simulink model "xpcserialbinarytest"  (Simulink 7.1)
settings: Solver=FixedStepDiscrete  StartTime=0.0  StopTime=inf  RelTol=1e-3
InitFcn:
  | trun = .1;
values from neighbouring files (symbols this model uses):
  count = count+1    (= 2)    [findVI.m]
undefined symbols (not defined in the file or in its folder): mquafifomask
libraries: xpclib x78, simulink x3
Description:
  | Serial Blocks Loopback Test Using Binary Encoding/Decoding
  | 
  | This model demonstrates the BINARY FIFO read block in a form that can be simulated without using any specific serial hardware.  The input to the FIFO write block is the concatenation of several pieces comprising two separate 'messages'.  The first message is the byte stream: [170, 1, N] and the second is [170 2 44 M] where N is an incrementing number and M is a decrementing number.  The initial '8' in the first constant is the number of elements that follow.  The '5' is an extraneous value that shows how the FIFO binary read will ignore extra information.
  | 
  | To run this test with real serial port hardware, replace the FIFO write block with the send/receive block with FIFO OUT that corresponds to your hardware from the xpclib rs232 section. Then feed the output signal back to the input with a wire to perform a loopback test.
settings Model: Creator=gweast  LastModifiedBy=Administrator  ExtModeArmWhenConnect=off  BufferReuse=off
settings OptimizationCC: BlockReduction=off  OptimizeBlockIOStorage=off  BufferReuse=off  ExpressionFolding=off  FoldNonRolledExpr=off  LocalBlockOutputs=off
settings DebuggingCC: SaveWithParameterizedLinksMsg=none  SignalResolutionControl=TryResolveAllWithWarning  MultiTaskDSMMsg=warning  MultiTaskCondExecSysMsg=none  StrictBusMsg=None
settings HardwareCC: ProdIntDivRoundTo=Zero  ProdEndianess=LittleEndian  ProdHWDeviceType=Generic->32-bit x86 compatible
settings RTWCC: SystemTargetFile=xpctarget.tlc  TemplateMakefile=xpc_default_tmf  Description=xPC Target  ProcessScript=xpctarget_make_rtw_hook  IncludeERTFirstTime=on
settings xpcTargetCC: TargetFcnLib=ansi_tfl_tmw.mat  TargetFunctionLibrary=ANSI_C  CompOptLevelCompliant=off  PortableWordSizes=off  xPCisDownloadable=off

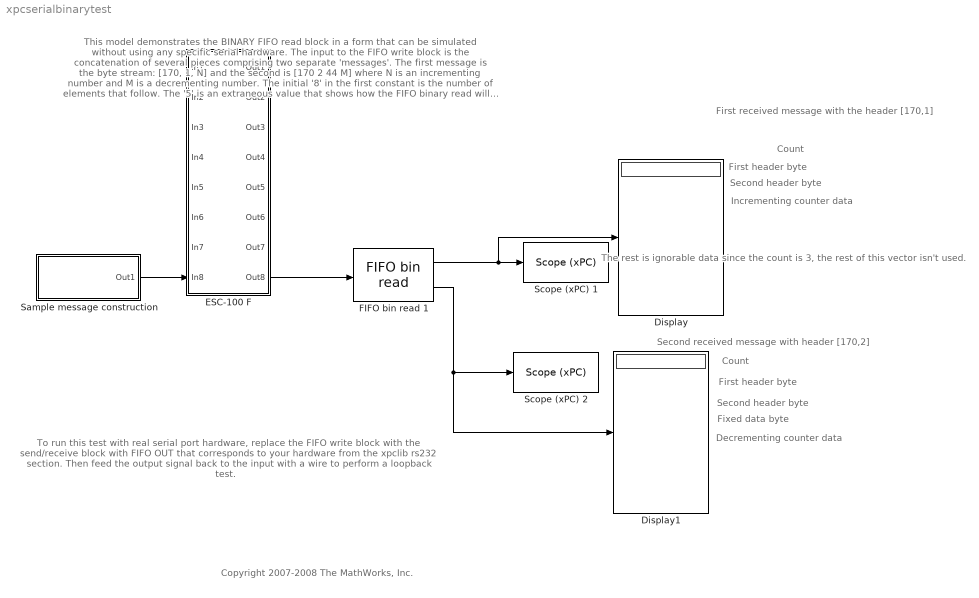
== system xpcserialbinarytest ==
  note: This model demonstrates the BINARY FIFO read block in a form that can
      | be simulated without using any specific serial hardware.  The input to
      | the FIFO write block is the concatenation of several pieces comprising
      | two separate 'messages'.  The first message is the byte stream:
      | [170, 1, N] and the second is [170 2 44 M] where N is an incrementing
      | number and M is a decrementing number.  The initial '8' in the first constant
      | is the number of elements that follow.  The '5' is an extraneous value that
      | shows how the FIFO binary read will ignore extra information.
  note: To run this test with
      | real serial port hardware,
      | replace the FIFO write
      | block with the send/receive
      | block with FIFO OUT that
      | corresponds to your
      | hardware from the xpclib
      | rs232 section. Then feed
      | the output signal back to
      | the input with a wire to
      | perform a loopback test.
  note: First received message
      | with the header [170,1]
  note: Count
  note: First header byte
  note: Second header byte
  note: Incrementing counter data
  note: The rest is ignorable
      | data since the count
      | is 3, the rest of this
      | vector isn't used.
  note: Count
  note: First header byte
  note: Second header byte
  note: Fixed data byte
  note: Decrementing counter data
  note: Second received message
      | with header [170,2]
  note: Copyright 2007-2008 The MathWorks, Inc.
  Display : Display
  Display1 : Display
  ESC-100 F : Subsystem  AncestorBlock=xpclib/RS232/Quatech/ESC-100/ESC-100 F  InitFcn=mquafifomask(3)  mask(ESC-100 RS232 Send Receive){group=Basic Setup, port=8, irqnum=10, slot=-1, baud1=115200, parity1=None, ndata1=8, nstop1=1, fifomode1=64 deep, rlevel1=half full, automode1=off, xmtfifosize1=1024, xmtdatatype1=count+16 bit int, rcvfifosize1=1024, baud2=115200, parity2=None, ndata2=8, nstop2=1, fifomode2=64 deep, rlevel2=half full, automode2=off, xmtfifosize2=1024, xmtdatatype2=8 bit uint null terminated, rcvfifosize2=1024, baud3=115200, parity3=None, ndata3=8, nstop3=1, fifomode3=64 deep, rlevel3=half full, automode3=on, xmtfifosize3=1024, xmtdatatype3=8 bit uint null terminated, rcvfifosize3=1024, buad4=115200, parity4=None, ndata4=8, nstop4=1, fifomode4=64 deep, rlevel4=half full, automode4=on, xmtfifosize4=1024, xmtdatatype4=8 bit uint null terminated, rcvfifosize4=1024, baud5=115200, parity5=None, ndata5=8, nstop5=1, fifomode5=64 deep, rlevel5=half full, automode5=on, xmtfifosize5=1024, xmtdatatype5=8 bit uint null terminated, rcvfifosize5=1024, baud6=115200, parity6=None, ndata6=8, nstop6=1, fifomode6=64 deep, rlevel6=half full, automode6=on, xmtfifosize6=1024, xmtdatatype6=8 bit uint null terminated, rcvfifosize6=1024, baud7=115200, parity7=None, ndata7=8, nstop7=1, fifomode7=64 deep, rlevel7=half full, automode7=on, xmtfifosize7=1024, xmtdatatype7=8 bit uint null terminated, rcvfifosize7=1024, baud8=57600, parity8=None, ndata8=8, nstop8=1, fifomode8=64 deep, rlevel8=quarter full, automode8=off, xmtfifosize8=1024, xmtdatatype8=count+16 bit int, rcvfifosize8=1024}
      mask prompts: group "Parameter group:"; port "Port to modify:"; irqnum "IRQ number:"; baud1 "Baud rate:"; parity1 "Parity:"; ndata1 "Data bits:"; nstop1 "Stop bits:"; fifomode1 "Hardware FIFO size:"; rlevel1 "Receive FIFO interrupt level:"; automode1 "Auto RTS/CTS:"; xmtfifosize1 "Transmit software FIFO size:"; xmtdatatype1 "Transmit FIFO data type:"; rcvfifosize1 "Receive software FIFO size:"; baud2 "Baud rate:"; parity2 "Parity:"; ndata2 "Data bits:"; nstop2 "Stop bits:"; fifomode2 "Hardware FIFO size:"; rlevel2 "Receive FIFO interrupt level:"; automode2 "Auto RTS/CTS:"; xmtfifosize2 "Transmit software FIFO size:"; xmtdatatype2 "Transmit fifo data type:"; rcvfifosize2 "Receive software FIFO size:"; baud3 "Baud rate:"; parity3 "Parity:"; ndata3 "Data bits:"; nstop3 "Stop bits:"; fifomode3 "Hardware FIFO size:"; rlevel3 "Receive FIFO interrupt level:"; automode3 "Auto RTS/CTS:"; xmtfifosize3 "Transmit software FIFO size:"; xmtdatatype3 "Transmit FIFO data type:"; rcvfifosize3 "Receive software FIFO size:"; buad4 "Baud rate:"; parity4 "Parity:"; ndata4 "Data bits:"; nstop4 "Stop bits:"; fifomode4 "Hardware FIFO size:"; rlevel4 "Receive FIFO interrupt level:"; automode4 "Auto RTS/CTS:"; xmtfifosize4 "Transmit software FIFO size:"; xmtdatatype4 "Transmit FIFO data type:"; rcvfifosize4 "Receive software FIFO size:"; baud5 "Baud rate:"; parity5 "Parity:"; ndata5 "Data bits:"; nstop5 "Stop bits:"; fifomode5 "Hardware FIFO size:"; rlevel5 "Receive FIFO interrupt level:"; automode5 "Auto RTS/CTS:"; xmtfifosize5 "Transmit software FIFO size:"; xmtdatatype5 "Transmit FIFO data type:"; rcvfifosize5 "Receive software FIFO size:"; baud6 "Baud rate:"; parity6 "Parity:"; ndata6 "Data bits:"; nstop6 "Stop bits:"; fifomode6 "Hardware FIFO size:"; rlevel6 "Receive FIFO interrupt level:"; automode6 "Auto RTS/CTS:"; xmtfifosize6 "Transmit software FIFO size:"; xmtdatatype6 "Transmit FIFO data type:"; rcvfifosize6 "Receive software fifo size:"; baud7 "Baud rate:"; parity7 "Parity:"; ndata7 "Data bits:"; nstop7 "Stop bits:"; fifomode7 "Hardware FIFO size:"; rlevel7 "Receive FIFO interrupt level:"; automode7 "Auto RTS/CTS:"; xmtfifosize7 "Transmit software FIFO size:"; xmtdatatype7 "Transmit FIFO data type:"; rcvfifosize7 "Receive software FIFO size:"; baud8 "Baud rate:"; parity8 "Parity:"; ndata8 "Data bits:"; nstop8 "Stop bits:"; fifomode8 "Hardware FIFO size:"; rlevel8 "Receive FIFO interrupt level:"; automode8 "Auto RTS/CTS:"; xmtfifosize8 "Transmit software FIFO size:"; xmtdatatype8 "Transmit FIFO data type:"; rcvfifosize8 "Receive software FIFO size:"
      mask help:
      | ESC-100
      | Quatech
      | RS232 Send Receive Subsystem
      mask init:
      | brdslot = slot;
      | mquafifomask( 1, 8, 1 );
      mask Help: helpview(fullfile(docroot, 'mapfiles', 'xpc.map'), 'Quatech_Subsystem')
      mask StyleString: popup(Board Setup|Basic Setup|FIFO Setup),popup(1|2|3|4|5|6|7|8),edit,edit,popup(921600|460800|230400|115200|57600|38400|19200|9600|4800|2400|1200|600|300|110),popup(None|Even|Odd|Mark|Space),popup(5|6|7|8),popup(1|2),popup(64 deep|16 deep|1 deep),popup(1|quarter full|half full|almost full),checkbox,edit,popup(count+32 bit int|count+32 bit uint|count+16 bit int|count+16 bit uint|8 bit int null terminated|8 bit uint null terminated),edit,popup(921600|460800|230400|115200|57600|38400|19200|9600|4800|2400|1200|600|300|110),popup(None|Even|Odd|Mark|Space),popup(5|6|7|8),popup(1|2),popup(64 deep|16 deep|1 deep),popup(1|quarter full|half full|almost full),checkbox,edit,popup(count+32 bit int|count+32 bit uint|count+16 bit int|count+16 bit uint|8 bit int null terminated|8 bit uint null terminated),edit,popup(921600|460800|230400|115200|57600|38400|19200|9600|4800|2400|1200|600|300|110),popup(None|Even|Odd|Mark|Space),popup(5|6|7|8),popup(1|2),popup(64 deep|16 deep|1 deep),popup(1|quarter full|half full|almost full),checkbox,edit,popup(count+32 bit int|count+32 bit uint|count+16 bit int|count+16 bit uint|8 bit int null terminated|8 bit uint null terminated),edit,popup(921600|460800|230400|115200|57600|38400|19200|9600|4800|2400|1200|600|300|110),popup(None|Even|Odd|Mark|Space),popup(5|6|7|8),popup(1|2),popup(64 deep|16 deep|1 deep),popup(1|quarter full|half full|almost full),checkbox,edit,popup(count+32 bit int|count+32 bit uint|count+16 bit int|count+16 bit uint|8 bit int null terminated|8 bit uint null terminated),edit,popup(921600|460800|230400|115200|57600|38400|19200|9600|4800|2400|1200|600|300|110),popup(None|Even|Odd|Mark|Space),popup(5|6|7|8),popup(1|2),popup(64 deep|16 deep|1 deep),popup(1|quarter full|half full|almost full),checkbox,edit,popup(count+32 bit int|count+32 bit uint|count+16 bit int|count+16 bit uint|8 bit int null terminated|8 bit uint null terminated),edit,popup(921600|460800|230400|115200|57600|38400|19200|9600|4800|2400|1200|600|300|110),popup(None|Even|Odd|Mark|Space),popup(5|6|7|8),popup(1|2),popup(64 deep|16 deep|1 deep),popup(1|quarter full|half full|almost full),checkbox,edit,popup(count+32 bit int|count+32 bit uint|count+16 bit int|count+16 bit uint|8 bit int null terminated|8 bit uint null terminated),edit,popup(921600|460800|230400|115200|57600|38400|19200|9600|4800|2400|1200|600|300|110),popup(None|Even|Odd|Mark|Space),popup(5|6|7|8),popup(1|2),popup(64 deep|16 deep|1 deep),popup(1|quarter full|half full|almost full),checkbox,edit,popup(count+32 bit int|count+32 bit uint|count+16 bit int|count+16 bit uint|8 bit int null terminated|8 bit uint null terminated),edit,popup(921600|460800|230400|115200|57600|38400|19200|9600|4800|2400|1200|600|300|110),popup(None|Even|Odd|Mark|Space),popup(5|6|7|8),popup(1|2),popup(64 deep|16 deep|1 deep),popup(1|quarter full|half full|almost full),checkbox,edit,popup(count+32 bit int|count+32 bit uint|count+16 bit int|count+16 bit uint|8 bit int null terminated|8 bit uint null terminated),edit
      mask CallbackString:
      | mquafifomask( 2, 8 );
      | |mquafifomask( 2, 8 );||||||||||||||||||||||||||||||||||||||||||||||||||||||||||||||||||||||||||||||||||
      mask Display:
      | disp('ESC-100\n\nRS232\n\nSend Receive\nFIFO OUT');
      | port_label( 'input', 1, 'XMT1' );
      | port_label( 'input', 2, 'XMT2' );
      | port_label( 'input', 3, 'XMT3' );
      | port_label( 'input', 4, 'XMT4' );
      | port_label( 'input', 5, 'XMT5' );
      | port_label( 'input', 6, 'XMT6' );
      | port_label( 'input', 7, 'XMT7' );
      | port_label( 'input', 8, 'XMT8' );
      | port_label( 'output', 1, 'FIFO1' );
      | port_label( 'output', 2, 'FIFO2' );
      | port_label( 'output', 3, 'FIFO3' );
      | port_label( 'output', 4, 'FIFO4' );
      | port_label( 'output', 5, 'FIFO5' );
      | port_label( 'output', 6, 'FIFO6' );
      | port_label( 'output', 7, 'FIFO7' );
      | port_label( 'output', 8, 'FIFO8' );
  FIFO bin read 1 : xpclib/RS232/FIFO bin read   header={char([170, 1]), char([170,2])}  lengths=[3 4]  hold=Zero output if no new data  enable=off  maxsize=6  outputtype=count+16 bit int  sampletime=trun
  Sample message construction : Subsystem
  Scope (xPC) 1 : xpclib/Misc./Scope (xPC)   SystemSampleTime=-1  scopeno=2  scopetype=Target  autostart=on  viewmode=Graphical sliding  formatstr='%15.6f'  grid=on  ylimits=[0,0]  nosamples=512  noprepostsamples=0  interleave=1  triggermode=FreeRun  triggersignal=1  triggerlevel=0.0  triggerslope=Either  triggerscope=1  triggersample=0  filename=data.dat  mode=Lazy  writesize=512  autorestart=off
  Scope (xPC) 2 : xpclib/Misc./Scope (xPC)   SystemSampleTime=-1  scopeno=1  scopetype=Target  autostart=on  viewmode=Graphical sliding  formatstr='%15.6f'  grid=on  ylimits=[0,0]  nosamples=512  noprepostsamples=0  interleave=1  triggermode=FreeRun  triggersignal=1  triggerlevel=0.0  triggerslope=Either  triggerscope=1  triggersample=0  filename=data.dat  mode=Lazy  writesize=512  autorestart=off
  wires:
  ESC-100 F/8(Out8) -> FIFO bin read 1/1
  Sample message construction/1(Out1) -> ESC-100 F/8(In8)
  FIFO bin read 1/1 -> Scope (xPC) 1/1, Display/1
  FIFO bin read 1/2 -> Scope (xPC) 2/1, Display1/1

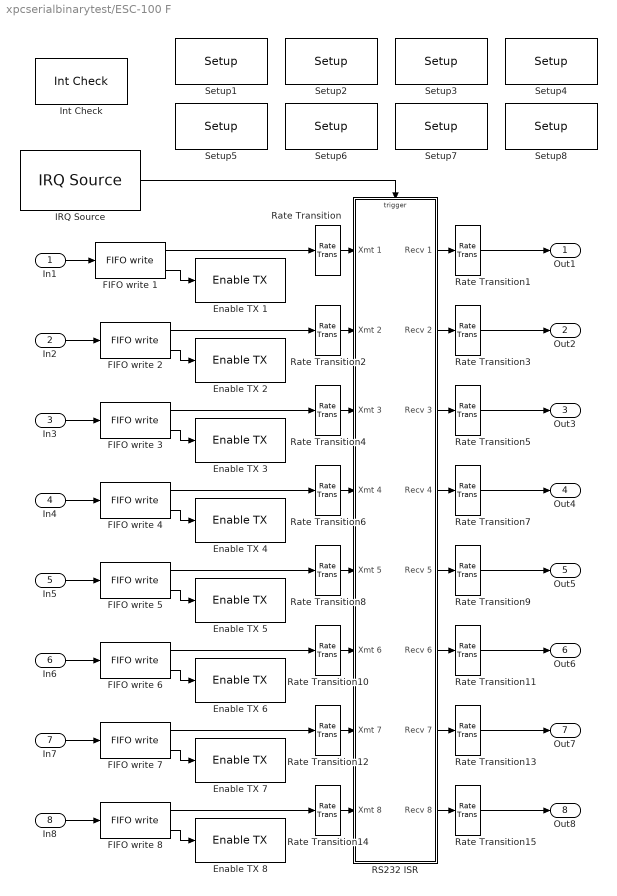
== system xpcserialbinarytest/ESC-100 F ==
  In1 : Inport  OutDataType=sfix(16)  OutScaling=2^0
  In2 : Inport  Port=2  OutDataType=sfix(16)  OutScaling=2^0
  In3 : Inport  Port=3  OutDataType=sfix(16)  OutScaling=2^0
  In4 : Inport  Port=4  OutDataType=sfix(16)  OutScaling=2^0
  In5 : Inport  Port=5  OutDataType=sfix(16)  OutScaling=2^0
  In6 : Inport  Port=6  OutDataType=sfix(16)  OutScaling=2^0
  In7 : Inport  Port=7  OutDataType=sfix(16)  OutScaling=2^0
  In8 : Inport  Port=8  OutDataType=sfix(16)  OutScaling=2^0
  Enable TX 1 : xpclib/RS232/Quatech/ESC-100/ESC-100 Internal blocks/Enable TX   port=1  slot=brdslot
  Enable TX 2 : xpclib/RS232/Quatech/ESC-100/ESC-100 Internal blocks/Enable TX   port=2  slot=brdslot
  Enable TX 3 : xpclib/RS232/Quatech/ESC-100/ESC-100 Internal blocks/Enable TX   port=3  slot=brdslot
  Enable TX 4 : xpclib/RS232/Quatech/ESC-100/ESC-100 Internal blocks/Enable TX   port=4  slot=brdslot
  Enable TX 5 : xpclib/RS232/Quatech/ESC-100/ESC-100 Internal blocks/Enable TX   port=5  slot=brdslot
  Enable TX 6 : xpclib/RS232/Quatech/ESC-100/ESC-100 Internal blocks/Enable TX   port=6  slot=brdslot
  Enable TX 7 : xpclib/RS232/Quatech/ESC-100/ESC-100 Internal blocks/Enable TX   port=7  slot=brdslot
  Enable TX 8 : xpclib/RS232/Quatech/ESC-100/ESC-100 Internal blocks/Enable TX   port=8  slot=brdslot
  FIFO write 1 : xpclib/RS232/FIFO write   size=1024  inputtype=count+16 bit int  present=on  sampletime=-1  id=XMT channel 1, IRQ 10
  FIFO write 2 : xpclib/RS232/FIFO write   size=1024  inputtype=8 bit uint null terminated  present=on  sampletime=-1  id=XMT channel 2, IRQ 10
  FIFO write 3 : xpclib/RS232/FIFO write   size=1024  inputtype=8 bit uint null terminated  present=on  sampletime=-1  id=XMT channel 3, IRQ 10
  FIFO write 4 : xpclib/RS232/FIFO write   size=1024  inputtype=8 bit uint null terminated  present=on  sampletime=-1  id=XMT channel 4, IRQ 10
  FIFO write 5 : xpclib/RS232/FIFO write   size=1024  inputtype=8 bit uint null terminated  present=on  sampletime=-1  id=XMT channel 5, IRQ 10
  FIFO write 6 : xpclib/RS232/FIFO write   size=1024  inputtype=8 bit uint null terminated  present=on  sampletime=-1  id=XMT channel 6, IRQ 10
  FIFO write 7 : xpclib/RS232/FIFO write   size=1024  inputtype=8 bit uint null terminated  present=on  sampletime=-1  id=XMT channel 7, IRQ 10
  FIFO write 8 : xpclib/RS232/FIFO write   size=1024  inputtype=count+16 bit int  present=on  sampletime=-1  id=XMT channel 8, IRQ 10
  IRQ Source : xpclib/Asynchronous Event/IRQ Source  irqNo=10  preempt=off  b_type=None/Other  slot=brdslot
  Int Check : xpclib/RS232/Quatech/ESC-100/ESC-100 Internal blocks/Int Check  slot=brdslot  irqnum=10
  RS232 ISR : Subsystem  TreatAsAtomicUnit=on  mask(RS232 ISR){slot=brdslot}
      mask help:
      | ESC-100
      | Quatech
      | Interrupt Service Routine
      mask init:
      | subslot = slot;
      mask Display:
      | disp('ESC-100\nISR');
      | port_label('input', 1, 'XMT1');
      | port_label('input', 2, 'XMT2');
      | port_label('input', 3, 'XMT3');
      | port_label('input', 4, 'XMT4');
      | port_label('input', 5, 'XMT5');
      | port_label('input', 6, 'XMT6');
      | port_label('input', 7, 'XMT7');
      | port_label('input', 8, 'XMT8');
      | port_label('output', 1, 'RCV1');
      | port_label('output', 2, 'RCV2');
      | port_label('output', 3, 'RCV3');
      | port_label('output', 4, 'RCV4');
      | port_label('output', 5, 'RCV5');
      | port_label('output', 6, 'RCV6');
      | port_label('output', 7, 'RCV7');
      | port_label('output', 8, 'RCV8');
  Rate Transition{,2,4,6,8,10,12} (7 alike) : RateTransition  Integrity=off  Deterministic=off
  Rate Transition{1,3,5,7,9,11,13,15} (8 alike) : RateTransition  Integrity=off  Deterministic=off  OutPortSampleTime=0
  Rate Transition14 : RateTransition  Integrity=off
  Setup1 : xpclib/RS232/Quatech/ESC-100/ESC-100 Internal blocks/Setup  port=1  baud=115200  width=8  nstop=1  parity=None  fmode=64 deep  rlevel=half full  ctsmode=off  slot=brdslot
  Setup2 : xpclib/RS232/Quatech/ESC-100/ESC-100 Internal blocks/Setup  port=2  baud=115200  width=8  nstop=1  parity=None  fmode=64 deep  rlevel=half full  ctsmode=off  slot=brdslot
  Setup3 : xpclib/RS232/Quatech/ESC-100/ESC-100 Internal blocks/Setup  port=3  baud=115200  width=8  nstop=1  parity=None  fmode=64 deep  rlevel=half full  ctsmode=on  slot=brdslot
  Setup4 : xpclib/RS232/Quatech/ESC-100/ESC-100 Internal blocks/Setup  port=4  baud=115200  width=8  nstop=1  parity=None  fmode=64 deep  rlevel=half full  ctsmode=on  slot=brdslot
  Setup5 : xpclib/RS232/Quatech/ESC-100/ESC-100 Internal blocks/Setup  port=5  baud=115200  width=8  nstop=1  parity=None  fmode=64 deep  rlevel=half full  ctsmode=on  slot=brdslot
  Setup6 : xpclib/RS232/Quatech/ESC-100/ESC-100 Internal blocks/Setup  port=6  baud=115200  width=8  nstop=1  parity=None  fmode=64 deep  rlevel=half full  ctsmode=on  slot=brdslot
  Setup7 : xpclib/RS232/Quatech/ESC-100/ESC-100 Internal blocks/Setup  port=7  baud=115200  width=8  nstop=1  parity=None  fmode=64 deep  rlevel=half full  ctsmode=on  slot=brdslot
  Setup8 : xpclib/RS232/Quatech/ESC-100/ESC-100 Internal blocks/Setup  port=8  baud=57600  width=8  nstop=1  parity=None  fmode=64 deep  rlevel=quarter full  ctsmode=off  slot=brdslot
  Out1 : Outport  OutDataType=sfix(16)  OutScaling=2^0
  Out2 : Outport  Port=2  OutDataType=sfix(16)  OutScaling=2^0
  Out3 : Outport  Port=3  OutDataType=sfix(16)  OutScaling=2^0
  Out4 : Outport  Port=4  OutDataType=sfix(16)  OutScaling=2^0
  Out5 : Outport  Port=5  OutDataType=sfix(16)  OutScaling=2^0
  Out6 : Outport  Port=6  OutDataType=sfix(16)  OutScaling=2^0
  Out7 : Outport  Port=7  OutDataType=sfix(16)  OutScaling=2^0
  Out8 : Outport  Port=8  OutDataType=sfix(16)  OutScaling=2^0
  wires:
  In8/1 -> FIFO write 8/1
  In7/1 -> FIFO write 7/1
  In6/1 -> FIFO write 6/1
  In5/1 -> FIFO write 5/1
  In4/1 -> FIFO write 4/1
  In3/1 -> FIFO write 3/1
  In2/1 -> FIFO write 2/1
  FIFO write 8/2 -> Enable TX 8/1
  FIFO write 7/2 -> Enable TX 7/1
  FIFO write 6/2 -> Enable TX 6/1
  FIFO write 5/2 -> Enable TX 5/1
  FIFO write 4/2 -> Enable TX 4/1
  FIFO write 3/2 -> Enable TX 3/1
  FIFO write 2/2 -> Enable TX 2/1
  FIFO write 8/1 -> Rate Transition14/1
  FIFO write 7/1 -> Rate Transition12/1
  FIFO write 6/1 -> Rate Transition10/1
  FIFO write 5/1 -> Rate Transition8/1
  FIFO write 4/1 -> Rate Transition6/1
  FIFO write 3/1 -> Rate Transition4/1
  FIFO write 2/1 -> Rate Transition2/1
  FIFO write 1/2 -> Enable TX 1/1
  FIFO write 1/1 -> Rate Transition/1
  In1/1 -> FIFO write 1/1
  IRQ Source/1 -> RS232 ISR/Trigger
  Rate Transition/1 -> RS232 ISR/1(Xmt 1)
  Rate Transition4/1 -> RS232 ISR/3(Xmt 3)
  Rate Transition6/1 -> RS232 ISR/4(Xmt 4)
  RS232 ISR/1(Recv 1) -> Rate Transition1/1
  RS232 ISR/2(Recv 2) -> Rate Transition3/1
  RS232 ISR/3(Recv 3) -> Rate Transition5/1
  Rate Transition1/1 -> Out1/1
  Rate Transition3/1 -> Out2/1
  Rate Transition5/1 -> Out3/1
  Rate Transition7/1 -> Out4/1
  Rate Transition2/1 -> RS232 ISR/2(Xmt 2)
  RS232 ISR/4(Recv 4) -> Rate Transition7/1
  Rate Transition14/1 -> RS232 ISR/8(Xmt 8)
  Rate Transition12/1 -> RS232 ISR/7(Xmt 7)
  Rate Transition10/1 -> RS232 ISR/6(Xmt 6)
  Rate Transition8/1 -> RS232 ISR/5(Xmt 5)
  Rate Transition9/1 -> Out5/1
  Rate Transition11/1 -> Out6/1
  Rate Transition13/1 -> Out7/1
  Rate Transition15/1 -> Out8/1
  RS232 ISR/5(Recv 5) -> Rate Transition9/1
  RS232 ISR/6(Recv 6) -> Rate Transition11/1
  RS232 ISR/7(Recv 7) -> Rate Transition13/1
  RS232 ISR/8(Recv 8) -> Rate Transition15/1

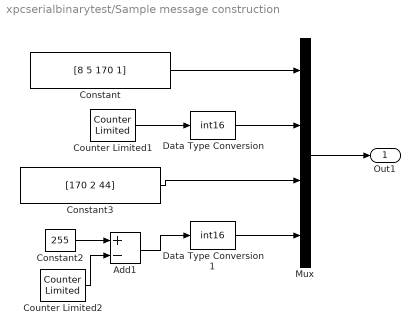
== system xpcserialbinarytest/Sample message construction ==
  Add1 : Sum  Inputs=+-  OutDataType=sfix(16)  OutScaling=2^-10
  Constant : Constant  Value=[8 5 170 1]  OutDataTypeMode=int16  OutDataType=sfix(16)  OutScaling=2^0  OutDataTypeStr=int16
  Constant2 : Constant  Value=255  OutDataType=sfix(16)  OutScaling=2^0
  Constant3 : Constant  Value=[170 2 44]  OutDataTypeMode=int16  OutDataType=sfix(16)  OutScaling=2^0  OutDataTypeStr=int16
  Counter Limited1 : simulink/Sources/Counter Limited  SystemSampleTime=-1  uplimit=255  tsamp=trun
  Counter Limited2 : simulink/Sources/Counter Limited  SystemSampleTime=-1  uplimit=255  tsamp=trun
  Data Type Conversion : DataTypeConversion  OutDataTypeMode=int16  OutDataType=sfix(16)  OutScaling=2^0  OutDataTypeStr=int16
  Data Type Conversion1 : DataTypeConversion  OutDataTypeMode=int16  OutDataType=sfix(16)  OutScaling=2^0  OutDataTypeStr=int16
  Mux : Mux
  Out1 : Outport  OutDataType=sfix(16)  OutScaling=2^0
  wires:
  Counter Limited1/1 -> Data Type Conversion/1
  Constant/1 -> Mux/1
  Constant3/1 -> Mux/3
  Data Type Conversion/1 -> Mux/2
  Data Type Conversion1/1 -> Mux/4
  Mux/1 -> Out1/1
  Constant2/1 -> Add1/1
  Counter Limited2/1 -> Add1/2
  Add1/1 -> Data Type Conversion1/1

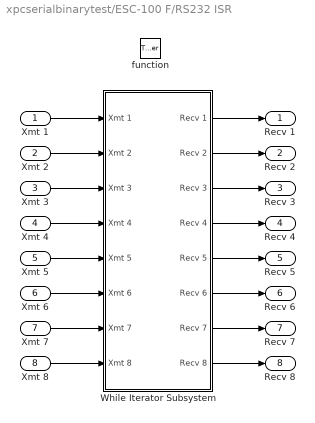
== system xpcserialbinarytest/ESC-100 F/RS232 ISR ==
  Xmt 1 : Inport  OutDataType=sfix(16)  OutScaling=2^0
  Xmt 2 : Inport  Port=2  OutDataType=sfix(16)  OutScaling=2^0
  Xmt 3 : Inport  Port=3  OutDataType=sfix(16)  OutScaling=2^0
  Xmt 4 : Inport  Port=4  OutDataType=sfix(16)  OutScaling=2^0
  Xmt 5 : Inport  Port=5  OutDataType=sfix(16)  OutScaling=2^0
  Xmt 6 : Inport  Port=6  OutDataType=sfix(16)  OutScaling=2^0
  Xmt 7 : Inport  Port=7  OutDataType=sfix(16)  OutScaling=2^0
  Xmt 8 : Inport  Port=8  OutDataType=sfix(16)  OutScaling=2^0
  function : TriggerPort  TriggerType=function-call
  While Iterator Subsystem : Subsystem  TreatAsAtomicUnit=on
  Recv 1 : Outport  OutDataType=sfix(16)  OutScaling=2^0
  Recv 2 : Outport  Port=2  OutDataType=sfix(16)  OutScaling=2^0
  Recv 3 : Outport  Port=3  OutDataType=sfix(16)  OutScaling=2^0
  Recv 4 : Outport  Port=4  OutDataType=sfix(16)  OutScaling=2^0
  Recv 5 : Outport  Port=5  OutDataType=sfix(16)  OutScaling=2^0
  Recv 6 : Outport  Port=6  OutDataType=sfix(16)  OutScaling=2^0
  Recv 7 : Outport  Port=7  OutDataType=sfix(16)  OutScaling=2^0
  Recv 8 : Outport  Port=8  OutDataType=sfix(16)  OutScaling=2^0
  wires:
  While Iterator Subsystem/8(Recv 8) -> Recv 8/1
  While Iterator Subsystem/7(Recv 7) -> Recv 7/1
  While Iterator Subsystem/6(Recv 6) -> Recv 6/1
  While Iterator Subsystem/5(Recv 5) -> Recv 5/1
  While Iterator Subsystem/4(Recv 4) -> Recv 4/1
  While Iterator Subsystem/3(Recv 3) -> Recv 3/1
  While Iterator Subsystem/2(Recv 2) -> Recv 2/1
  While Iterator Subsystem/1(Recv 1) -> Recv 1/1
  Xmt 8/1 -> While Iterator Subsystem/8(Xmt 8)
  Xmt 7/1 -> While Iterator Subsystem/7(Xmt 7)
  Xmt 6/1 -> While Iterator Subsystem/6(Xmt 6)
  Xmt 5/1 -> While Iterator Subsystem/5(Xmt 5)
  Xmt 4/1 -> While Iterator Subsystem/4(Xmt 4)
  Xmt 3/1 -> While Iterator Subsystem/3(Xmt 3)
  Xmt 2/1 -> While Iterator Subsystem/2(Xmt 2)
  Xmt 1/1 -> While Iterator Subsystem/1(Xmt 1)

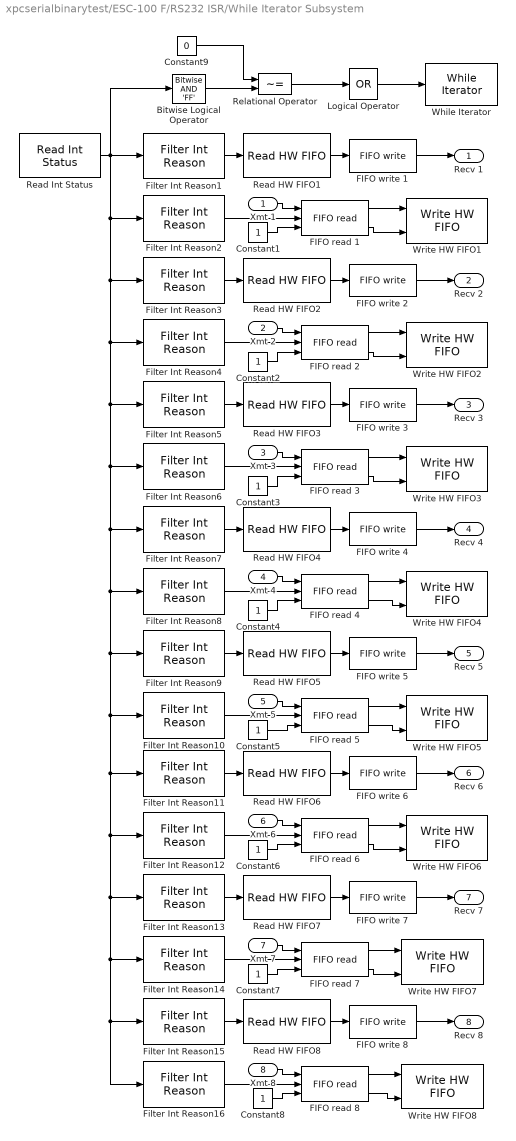
== system xpcserialbinarytest/ESC-100 F/RS232 ISR/While Iterator Subsystem ==
  Xmt 1 : Inport  OutDataType=sfix(16)  OutScaling=2^0
  Xmt 2 : Inport  Port=2  OutDataType=sfix(16)  OutScaling=2^0
  Xmt 3 : Inport  Port=3  OutDataType=sfix(16)  OutScaling=2^0
  Xmt 4 : Inport  Port=4  OutDataType=sfix(16)  OutScaling=2^0
  Xmt 5 : Inport  Port=5  OutDataType=sfix(16)  OutScaling=2^0
  Xmt 6 : Inport  Port=6  OutDataType=sfix(16)  OutScaling=2^0
  Xmt 7 : Inport  Port=7  OutDataType=sfix(16)  OutScaling=2^0
  Xmt 8 : Inport  Port=8  OutDataType=sfix(16)  OutScaling=2^0
  Bitwise Logical Operator : simulink/Logic and Bit Operations/Bitwise Operator  logicop=AND  UseBitMask=on  BitMask='FF'  BitMaskRealWorld=Stored Integer
  Constant{1..8} (8 alike) : Constant  OutDataTypeMode=uint32  OutDataType=sfix(16)  OutScaling=2^0  OutDataTypeStr=uint32
  Constant9 : Constant  Value=0  OutDataTypeMode=uint32  OutDataType=sfix(16)  OutScaling=2^0  OutDataTypeStr=uint32
  FIFO read {1..8} (8 alike) : xpclib/RS232/FIFO read   maxsize=60  minsize=1  usedelimiter=off  delimiter=13  outputtype=count+32 bit uint  enable=on  enableout=on  sampletime=-1
  FIFO write 1 : xpclib/RS232/FIFO write   size=1024  inputtype=count+32 bit uint  present=off  sampletime=-1  id=RCV channel 1, IRQ 10
  FIFO write 2 : xpclib/RS232/FIFO write   size=1024  inputtype=count+32 bit uint  present=off  sampletime=-1  id=RCV channel 2, IRQ 10
  FIFO write 3 : xpclib/RS232/FIFO write   size=1024  inputtype=count+32 bit uint  present=off  sampletime=-1  id=RCV channel 3, IRQ 10
  FIFO write 4 : xpclib/RS232/FIFO write   size=1024  inputtype=count+32 bit uint  present=off  sampletime=-1  id=RCV channel 4, IRQ 10
  FIFO write 5 : xpclib/RS232/FIFO write   size=1024  inputtype=count+32 bit uint  present=off  sampletime=-1  id=RCV channel 5, IRQ 10
  FIFO write 6 : xpclib/RS232/FIFO write   size=1024  inputtype=count+32 bit uint  present=off  sampletime=-1  id=RCV channel 6, IRQ 10
  FIFO write 7 : xpclib/RS232/FIFO write   size=1024  inputtype=count+32 bit uint  present=off  sampletime=-1  id=RCV channel 7, IRQ 10
  FIFO write 8 : xpclib/RS232/FIFO write   size=1024  inputtype=count+32 bit uint  present=off  sampletime=-1  id=RCV channel 8, IRQ 10
  Filter Int Reason1 : xpclib/RS232/Quatech/ESC-100/ESC-100 Internal blocks/Filter Int Reason  port=1  value=Receive data
  Filter Int Reason10 : xpclib/RS232/Quatech/ESC-100/ESC-100 Internal blocks/Filter Int Reason  port=5  value=Transmitter empty
  Filter Int Reason11 : xpclib/RS232/Quatech/ESC-100/ESC-100 Internal blocks/Filter Int Reason  port=6  value=Receive data
  Filter Int Reason12 : xpclib/RS232/Quatech/ESC-100/ESC-100 Internal blocks/Filter Int Reason  port=6  value=Transmitter empty
  Filter Int Reason13 : xpclib/RS232/Quatech/ESC-100/ESC-100 Internal blocks/Filter Int Reason  port=7  value=Receive data
  Filter Int Reason14 : xpclib/RS232/Quatech/ESC-100/ESC-100 Internal blocks/Filter Int Reason  port=7  value=Transmitter empty
  Filter Int Reason15 : xpclib/RS232/Quatech/ESC-100/ESC-100 Internal blocks/Filter Int Reason  port=8  value=Receive data
  Filter Int Reason16 : xpclib/RS232/Quatech/ESC-100/ESC-100 Internal blocks/Filter Int Reason  port=8  value=Transmitter empty
  Filter Int Reason2 : xpclib/RS232/Quatech/ESC-100/ESC-100 Internal blocks/Filter Int Reason  port=1  value=Transmitter empty
  Filter Int Reason3 : xpclib/RS232/Quatech/ESC-100/ESC-100 Internal blocks/Filter Int Reason  port=2  value=Receive data
  Filter Int Reason4 : xpclib/RS232/Quatech/ESC-100/ESC-100 Internal blocks/Filter Int Reason  port=2  value=Transmitter empty
  Filter Int Reason5 : xpclib/RS232/Quatech/ESC-100/ESC-100 Internal blocks/Filter Int Reason  port=3  value=Receive data
  Filter Int Reason6 : xpclib/RS232/Quatech/ESC-100/ESC-100 Internal blocks/Filter Int Reason  port=3  value=Transmitter empty
  Filter Int Reason7 : xpclib/RS232/Quatech/ESC-100/ESC-100 Internal blocks/Filter Int Reason  port=4  value=Receive data
  Filter Int Reason8 : xpclib/RS232/Quatech/ESC-100/ESC-100 Internal blocks/Filter Int Reason  port=4  value=Transmitter empty
  Filter Int Reason9 : xpclib/RS232/Quatech/ESC-100/ESC-100 Internal blocks/Filter Int Reason  port=5  value=Receive data
  Logical Operator : Logic  Operator=OR  Inputs=1  AllPortsSameDT=off
  Read HW FIFO1 : xpclib/RS232/Quatech/ESC-100/ESC-100 Internal blocks/Read HW FIFO  port=1  flush=on  slot=subslot
  Read HW FIFO2 : xpclib/RS232/Quatech/ESC-100/ESC-100 Internal blocks/Read HW FIFO  port=2  flush=on  slot=subslot
  Read HW FIFO3 : xpclib/RS232/Quatech/ESC-100/ESC-100 Internal blocks/Read HW FIFO  port=3  flush=on  slot=subslot
  Read HW FIFO4 : xpclib/RS232/Quatech/ESC-100/ESC-100 Internal blocks/Read HW FIFO  port=4  flush=on  slot=subslot
  Read HW FIFO5 : xpclib/RS232/Quatech/ESC-100/ESC-100 Internal blocks/Read HW FIFO  port=5  flush=on  slot=subslot
  Read HW FIFO6 : xpclib/RS232/Quatech/ESC-100/ESC-100 Internal blocks/Read HW FIFO  port=6  flush=on  slot=subslot
  Read HW FIFO7 : xpclib/RS232/Quatech/ESC-100/ESC-100 Internal blocks/Read HW FIFO  port=7  flush=on  slot=subslot
  Read HW FIFO8 : xpclib/RS232/Quatech/ESC-100/ESC-100 Internal blocks/Read HW FIFO  port=8  flush=on  slot=subslot
  Read Int Status : xpclib/RS232/Quatech/ESC-100/ESC-100 Internal blocks/Read Int Status  slot=subslot
  Relational Operator : RelationalOperator  Operator=~=
  While Iterator : WhileIterator  MaxIters=65  WhileBlockType=do-while
  Write HW FIFO1 : xpclib/RS232/Quatech/ESC-100/ESC-100 Internal blocks/Write HW FIFO  port=1  slot=subslot
  Write HW FIFO2 : xpclib/RS232/Quatech/ESC-100/ESC-100 Internal blocks/Write HW FIFO  port=2  slot=subslot
  Write HW FIFO3 : xpclib/RS232/Quatech/ESC-100/ESC-100 Internal blocks/Write HW FIFO  port=3  slot=subslot
  Write HW FIFO4 : xpclib/RS232/Quatech/ESC-100/ESC-100 Internal blocks/Write HW FIFO  port=4  slot=subslot
  Write HW FIFO5 : xpclib/RS232/Quatech/ESC-100/ESC-100 Internal blocks/Write HW FIFO  port=5  slot=subslot
  Write HW FIFO6 : xpclib/RS232/Quatech/ESC-100/ESC-100 Internal blocks/Write HW FIFO  port=6  slot=subslot
  Write HW FIFO7 : xpclib/RS232/Quatech/ESC-100/ESC-100 Internal blocks/Write HW FIFO  port=7  slot=subslot
  Write HW FIFO8 : xpclib/RS232/Quatech/ESC-100/ESC-100 Internal blocks/Write HW FIFO  port=8  slot=subslot
  Recv 1 : Outport  OutDataType=sfix(16)  OutScaling=2^0
  Recv 2 : Outport  Port=2  OutDataType=sfix(16)  OutScaling=2^0
  Recv 3 : Outport  Port=3  OutDataType=sfix(16)  OutScaling=2^0
  Recv 4 : Outport  Port=4  OutDataType=sfix(16)  OutScaling=2^0
  Recv 5 : Outport  Port=5  OutDataType=sfix(16)  OutScaling=2^0
  Recv 6 : Outport  Port=6  OutDataType=sfix(16)  OutScaling=2^0
  Recv 7 : Outport  Port=7  OutDataType=sfix(16)  OutScaling=2^0
  Recv 8 : Outport  Port=8  OutDataType=sfix(16)  OutScaling=2^0
  wires:
  Constant9/1 -> Relational Operator/1
  Bitwise Logical Operator/1 -> Relational Operator/2
  Relational Operator/1 -> Logical Operator/1
  Logical Operator/1 -> While Iterator/1
  Constant8/1 -> FIFO read 8/3
  Constant7/1 -> FIFO read 7/3
  Constant6/1 -> FIFO read 6/3
  Constant5/1 -> FIFO read 5/3
  Constant4/1 -> FIFO read 4/3
  Constant3/1 -> FIFO read 3/3
  Constant2/1 -> FIFO read 2/3
  Constant1/1 -> FIFO read 1/3
  FIFO read 1/2 -> Write HW FIFO1/2
  FIFO read 1/1 -> Write HW FIFO1/1
  FIFO read 2/2 -> Write HW FIFO2/2
  FIFO read 2/1 -> Write HW FIFO2/1
  FIFO read 3/2 -> Write HW FIFO3/2
  FIFO read 3/1 -> Write HW FIFO3/1
  FIFO read 4/2 -> Write HW FIFO4/2
  FIFO read 4/1 -> Write HW FIFO4/1
  FIFO read 5/2 -> Write HW FIFO5/2
  FIFO read 5/1 -> Write HW FIFO5/1
  FIFO read 6/2 -> Write HW FIFO6/2
  FIFO read 6/1 -> Write HW FIFO6/1
  FIFO read 7/2 -> Write HW FIFO7/2
  FIFO read 7/1 -> Write HW FIFO7/1
  FIFO read 8/2 -> Write HW FIFO8/2
  FIFO read 8/1 -> Write HW FIFO8/1
  Xmt 8/1 -> FIFO read 8/1
  Filter Int Reason16/1 -> FIFO read 8/2
  Read HW FIFO8/1 -> FIFO write 8/1
  FIFO write 8/1 -> Recv 8/1
  Filter Int Reason15/1 -> Read HW FIFO8/1
  Xmt 7/1 -> FIFO read 7/1
  Filter Int Reason14/1 -> FIFO read 7/2
  Read HW FIFO7/1 -> FIFO write 7/1
  FIFO write 7/1 -> Recv 7/1
  Filter Int Reason13/1 -> Read HW FIFO7/1
  Xmt 6/1 -> FIFO read 6/1
  Filter Int Reason12/1 -> FIFO read 6/2
  Read HW FIFO6/1 -> FIFO write 6/1
  FIFO write 6/1 -> Recv 6/1
  Filter Int Reason11/1 -> Read HW FIFO6/1
  Xmt 5/1 -> FIFO read 5/1
  Filter Int Reason10/1 -> FIFO read 5/2
  Read HW FIFO5/1 -> FIFO write 5/1
  FIFO write 5/1 -> Recv 5/1
  Filter Int Reason9/1 -> Read HW FIFO5/1
  Xmt 4/1 -> FIFO read 4/1
  Filter Int Reason8/1 -> FIFO read 4/2
  Read HW FIFO4/1 -> FIFO write 4/1
  FIFO write 4/1 -> Recv 4/1
  Filter Int Reason7/1 -> Read HW FIFO4/1
  Xmt 3/1 -> FIFO read 3/1
  Filter Int Reason6/1 -> FIFO read 3/2
  Read HW FIFO3/1 -> FIFO write 3/1
  FIFO write 3/1 -> Recv 3/1
  Filter Int Reason5/1 -> Read HW FIFO3/1
  Xmt 2/1 -> FIFO read 2/1
  Filter Int Reason4/1 -> FIFO read 2/2
  Read HW FIFO2/1 -> FIFO write 2/1
  FIFO write 2/1 -> Recv 2/1
  Filter Int Reason3/1 -> Read HW FIFO2/1
  Xmt 1/1 -> FIFO read 1/1
  Filter Int Reason2/1 -> FIFO read 1/2
  Read HW FIFO1/1 -> FIFO write 1/1
  FIFO write 1/1 -> Recv 1/1
  Filter Int Reason1/1 -> Read HW FIFO1/1
  Read Int Status/1 -> Bitwise Logical Operator/1, Filter Int Reason15/1, Filter Int Reason16/1, Filter Int Reason14/1, Filter Int Reason13/1, Filter Int Reason12/1, Filter Int Reason11/1, Filter Int Reason10/1, Filter Int Reason9/1, Filter Int Reason8/1, Filter Int Reason7/1, Filter Int Reason6/1, Filter Int Reason5/1, Filter Int Reason4/1, Filter Int Reason3/1, Filter Int Reason2/1, Filter Int Reason1/1
